simulink model "observer"  (R2021a)
settings: Solver=VariableStepAuto  StartTime=0.0  StopTime=20  RelTol=1e-3
values from neighbouring files (symbols this model uses):
  B = [ b11,b12 ... (first row only)    [Linearmodel.m]    (also in matlab.mat = [0 1])
  K = lqr(A,B,Q,R)    [Linearmodel.m]    (also in matlab.mat = [20 20])
  L = Rmat2RPY(R)*180/pi    [NLT2.m]    (also in Rmat2PRY.m = [phi;theta;psi]; matlab.mat = [2 4])
settings Model: Creator=Sirius  LastModifiedBy=Sirius

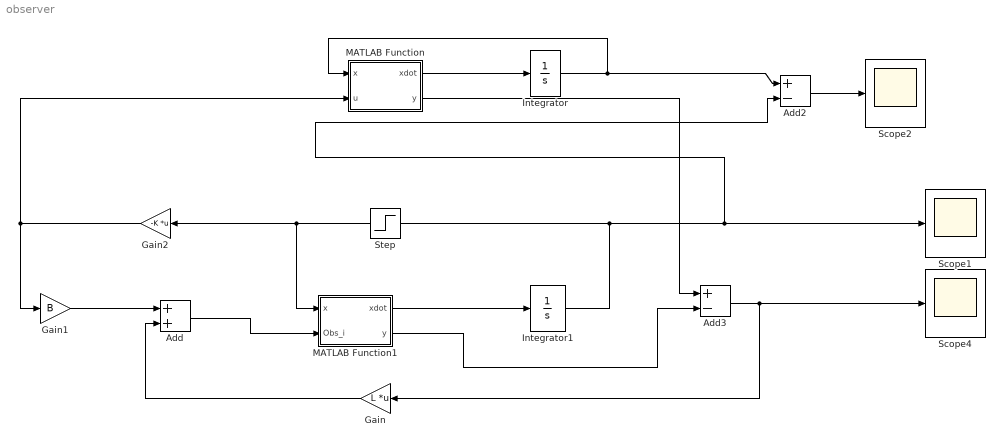
== system observer ==
  Add : Sum
  Add2 : Sum  Inputs=+-
  Add3 : Sum  Inputs=+-
  Gain : Gain  Gain=L  Multiplication=Matrix(K*u)
  Gain1 : Gain  Gain=B
  Gain2 : Gain  Gain=-K  Multiplication=Matrix(K*u)
  Integrator : Integrator  InitialCondition=[10;2]
  Integrator1 : Integrator  InitialCondition=[0;0]
  MATLAB Function : MATLAB Function  TreatAsAtomicUnit=on
  MATLAB Function1 : MATLAB Function  TreatAsAtomicUnit=on
  Scope1 : Scope
  Scope2 : Scope
  Scope4 : Scope
  Step : Step  SampleTime=0
  wires:
  MATLAB Function/1(xdot) -> Integrator/1
  Integrator/1 -> MATLAB Function/1(x), Add2/1
  Add/1 -> MATLAB Function1/2(Obs_i)
  MATLAB Function1/1(xdot) -> Integrator1/1
  Integrator1/1 -> Add2/2, Scope1/1, Gain2/1, MATLAB Function1/1(x)
  MATLAB Function1/2(y) -> Add3/2
  Add3/1 -> Scope4/1, Gain/1
  Gain1/1 -> Add/1
  Gain/1 -> Add/2
  Gain2/1 -> MATLAB Function/2(u), Gain1/1
  Add2/1 -> Scope2/1
  MATLAB Function/2(y) -> Add3/1

== matlab function observer/MATLAB Function ==
  data: x input; xdot output; u input; y output
function [xdot,y] = Sys(x,u)
A=[-1,1;0,1];
B=[0;1];
C=[1,0];
D=0;
xdot=A*x+B*u;
y=C*x+D*u;
end

== matlab function observer/MATLAB Function1 ==
  data: x input; xdot output; Obs_i input; y output
function [xdot,y] = Sys(x,Obs_i)
A=[-1,1;0,1];
B=[0;1];
C=[1,0];
D=0;
xdot=A*x+Obs_i;
y=C*x;
end
